simulink model "Parabolas - copia"  (R2018a)
settings: Solver=VariableStepAuto  StartTime=0.0  StopTime=10.0  RelTol=1e-3
values from neighbouring files (symbols this model uses):
  alt = alturas(2)    [Parabola - copia.m]    (also in Parabola.m = alturas(altura+1); Parabola_Seguridad.m = alturas(altura+1))
  ang = 0*pi/12    (= 0)    [Parabola - copia.m]    (also in Parabola.m = -0.523598775598; Parabola_Seguridad.m = 0.389)
  x = x + V*t + 0.5*ace*t^2    (= 0)    [Parabola - copia.m]    (also in Parabola.m = caida(dif,altura,1); Parabola_Seguridad.m = -0.25:0.01:0.25; linea.m = -0.25:0.01:0.25)
undefined symbols (not defined in the file or in its folder): magnitude
settings Model: Creator=Carlos  LastModifiedBy=Carlos

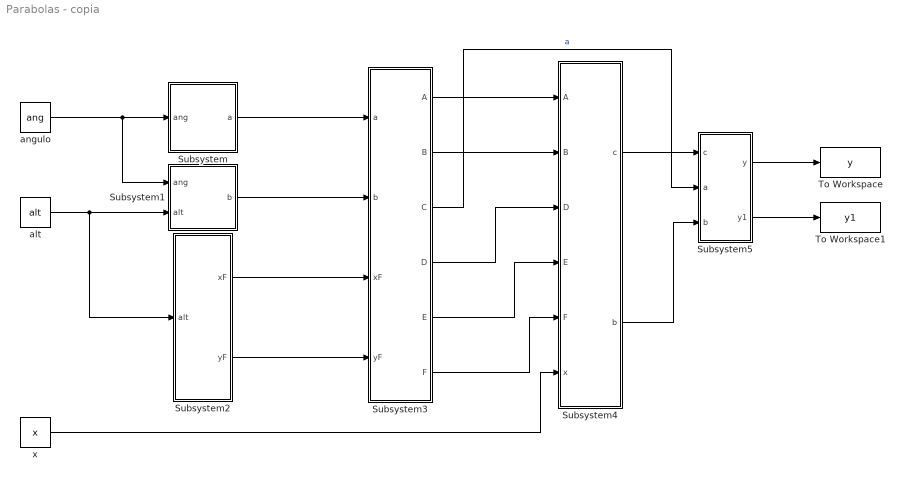
== system Parabolas - copia ==
  Subsystem : Subsystem
  Subsystem1 : Subsystem
  Subsystem2 : Subsystem
  Subsystem3 : Subsystem
  Subsystem4 : Subsystem
  Subsystem5 : Subsystem
  To Workspace : ToWorkspace  VariableName=y  SampleTime=-1
  To Workspace1 : ToWorkspace  VariableName=y1  SampleTime=-1
  alt : Constant  Value=alt
  angulo : Constant  Value=ang
  x : Constant  Value=x
  wires:
  angulo/1 -> Subsystem1/1(ang), Subsystem/1(ang)
  alt/1 -> Subsystem2/1("alt "), Subsystem1/2(alt)
  Subsystem/1(a) -> Subsystem3/1(a)
  Subsystem1/1(b) -> Subsystem3/2(b)
  Subsystem2/1(xF) -> Subsystem3/3(xF)
  Subsystem2/2(yF) -> Subsystem3/4(yF)
  Subsystem3/1(A) -> Subsystem4/1(A)
  Subsystem3/2(B) -> Subsystem4/2(B)
  Subsystem3/4(D) -> Subsystem4/3(D)
  Subsystem3/5(E) -> Subsystem4/4(E)
  x/1 -> Subsystem4/6(x)
  Subsystem3/6(F) -> Subsystem4/5(F)
  Subsystem4/1(c) -> Subsystem5/1(c)
  Subsystem3/3(C) -> Subsystem5/2(a)  "a"
  Subsystem4/2(b) -> Subsystem5/3(b)
  Subsystem5/1(y) -> To Workspace/1
  Subsystem5/2(y1) -> To Workspace1/1

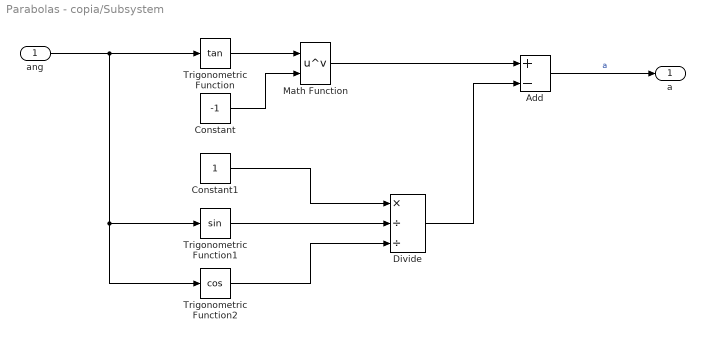
== system Parabolas - copia/Subsystem ==
  ang : Inport
  Add : Sum  Inputs=+-
  Constant : Constant  Value=-1
  Constant1 : Constant
  Divide : Product  Inputs=*//
  Math Function : Math  Operator=pow  SaturateOnIntegerOverflow=on
  Trigonometric Function : Trigonometry  Operator=tan
  Trigonometric Function1 : Trigonometry
  Trigonometric Function2 : Trigonometry  Operator=cos
  a : Outport
  wires:
  Trigonometric Function/1 -> Math Function/1
  Trigonometric Function1/1 -> Divide/2
  Trigonometric Function2/1 -> Divide/3
  ang/1 -> Trigonometric Function2/1, Trigonometric Function1/1, Trigonometric Function/1
  Constant1/1 -> Divide/1
  Math Function/1 -> Add/1
  Divide/1 -> Add/2
  Add/1 -> a/1  "a"
  Constant/1 -> Math Function/2

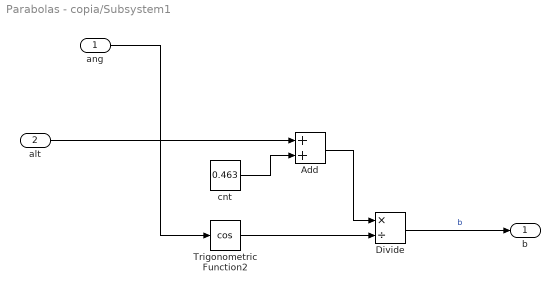
== system Parabolas - copia/Subsystem1 ==
  ang : Inport
  alt : Inport  Port=2
  Add : Sum
  Divide : Product  Inputs=*/
  Trigonometric Function2 : Trigonometry  Operator=cos
  cnt : Constant  Value=0.463
  b : Outport
  wires:
  Divide/1 -> b/1  "b"
  Trigonometric Function2/1 -> Divide/2
  Add/1 -> Divide/1
  alt/1 -> Add/1
  cnt/1 -> Add/2
  ang/1 -> Trigonometric Function2/1

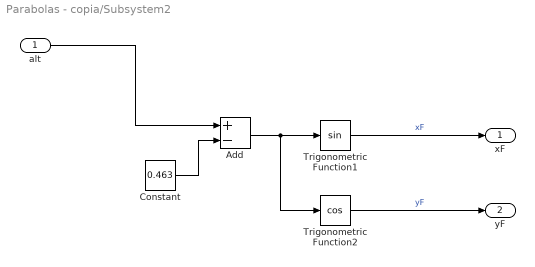
== system Parabolas - copia/Subsystem2 ==
  "alt " : Inport
  Add : Sum  Inputs=+-
  Constant : Constant  Value=0.463
  Trigonometric Function1 : Trigonometry
  Trigonometric Function2 : Trigonometry  Operator=cos
  xF : Outport
  yF : Outport  Port=2
  wires:
  Trigonometric Function1/1 -> xF/1  "xF"
  Constant/1 -> Add/2
  "alt "/1 -> Add/1
  Add/1 -> Trigonometric Function2/1, Trigonometric Function1/1
  Trigonometric Function2/1 -> yF/1  "yF"

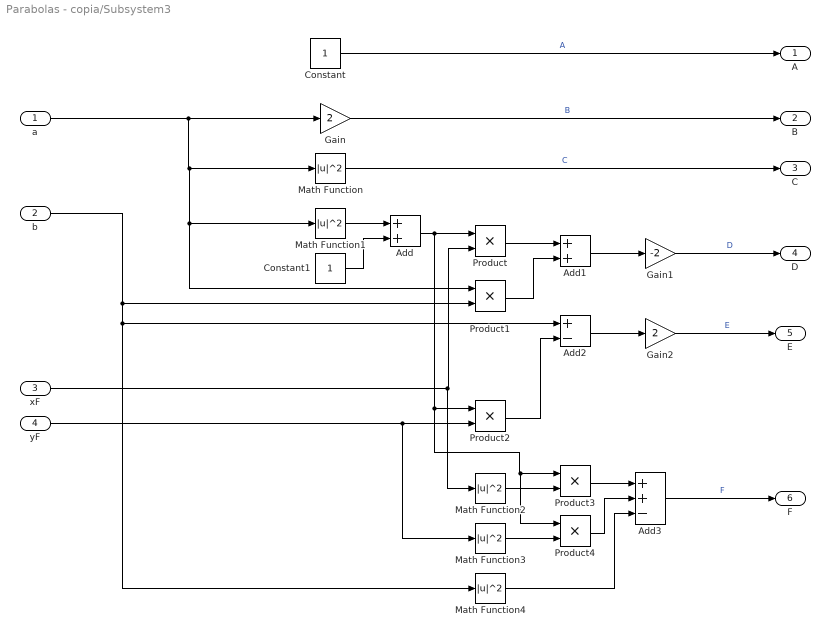
== system Parabolas - copia/Subsystem3 ==
  a : Inport
  b : Inport  Port=2
  xF : Inport  Port=3
  yF : Inport  Port=4
  Add : Sum
  Add1 : Sum
  Add2 : Sum  Inputs=+-
  Add3 : Sum  Inputs=++-
  Constant : Constant
  Constant1 : Constant
  Gain : Gain  Gain=2
  Gain1 : Gain  Gain=-2
  Gain2 : Gain  Gain=2
  Math Function{,1..4} (5 alike) : Math  Operator=magnitude^2  SaturateOnIntegerOverflow=on
  Product{,1..4} (5 alike) : Product
  A : Outport
  B : Outport  Port=2
  C : Outport  Port=3
  D : Outport  Port=4
  E : Outport  Port=5
  F : Outport  Port=6
  wires:
  Math Function3/1 -> Product4/2
  Gain1/1 -> D/1  "D"
  Add/1 -> Product4/1, Product3/1, Product2/1, Product/1
  Product4/1 -> Add3/2
  Product2/1 -> Add2/2
  Constant1/1 -> Add/2
  a/1 -> Product1/1, Math Function1/1, Math Function/1, Gain/1
  Math Function/1 -> C/1  "C"
  b/1 -> Math Function4/1, Add2/1, Product1/2
  Add1/1 -> Gain1/1
  xF/1 -> Math Function2/1, Product/2
  Math Function1/1 -> Add/1
  Add2/1 -> Gain2/1
  Product/1 -> Add1/1
  Math Function2/1 -> Product3/2
  Gain/1 -> B/1  "B"
  Product1/1 -> Add1/2
  yF/1 -> Math Function3/1, Product2/2
  Math Function4/1 -> Add3/3
  Product3/1 -> Add3/1
  Gain2/1 -> E/1  "E"
  Add3/1 -> F/1  "F"
  Constant/1 -> A/1  "A"

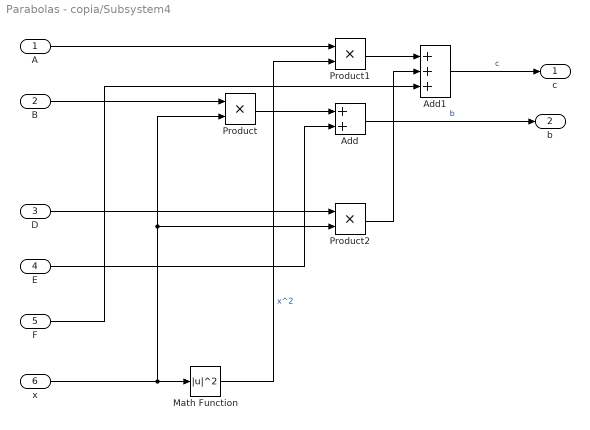
== system Parabolas - copia/Subsystem4 ==
  A : Inport
  B : Inport  Port=2
  D : Inport  Port=3
  E : Inport  Port=4
  F : Inport  Port=5
  x : Inport  Port=6
  Add : Sum
  Add1 : Sum  Inputs=+++
  Math Function : Math  Operator=magnitude^2  SaturateOnIntegerOverflow=on
  Product : Product
  Product1 : Product
  Product2 : Product
  c : Outport
  b : Outport  Port=2
  wires:
  A/1 -> Product1/1
  Product2/1 -> Add1/2
  x/1 -> Product2/2, Product/2, Math Function/1
  Product/1 -> Add/1
  Add1/1 -> c/1  "c"
  Add/1 -> b/1  "b"
  Math Function/1 -> Product1/2  "x^2"
  Product1/1 -> Add1/1
  E/1 -> Add/2
  D/1 -> Product2/1
  B/1 -> Product/1
  F/1 -> Add1/3

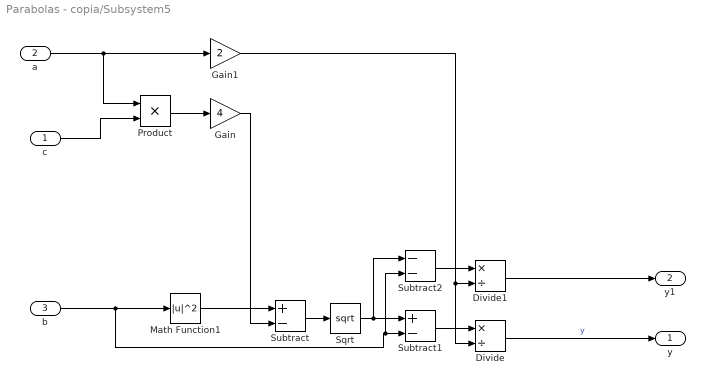
== system Parabolas - copia/Subsystem5 ==
  c : Inport
  a : Inport  Port=2
  b : Inport  Port=3
  Divide : Product  Inputs=*/
  Divide1 : Product  Inputs=*/
  Gain : Gain  Gain=4
  Gain1 : Gain  Gain=2
  Math Function1 : Math  Operator=magnitude^2  SaturateOnIntegerOverflow=on
  Product : Product
  Sqrt : Sqrt  SaturateOnIntegerOverflow=on
  Subtract : Sum  Inputs=+-
  Subtract1 : Sum  Inputs=+-
  Subtract2 : Sum  Inputs=--
  y : Outport
  y1 : Outport  Port=2
  wires:
  Sqrt/1 -> Subtract2/1, Subtract1/1
  Subtract/1 -> Sqrt/1
  a/1 -> Gain1/1, Product/1
  Subtract1/1 -> Divide/1
  Product/1 -> Gain/1
  b/1 -> Subtract2/2, Subtract1/2, Math Function1/1
  Gain/1 -> Subtract/2
  Gain1/1 -> Divide1/2, Divide/2
  Math Function1/1 -> Subtract/1
  Divide/1 -> y/1  "y"
  c/1 -> Product/2
  Subtract2/1 -> Divide1/1
  Divide1/1 -> y1/1
